simulink model "LCK"  (R2018b)
settings: Solver=FixedStepDiscrete  StartTime=0.0  StopTime=inf  FixedStep=0.01  RelTol=1e-3
PostLoadFcn:
  | if any(exist('dsrtsu_mdlpostloadfcn', 'file') ~= 0), dsrtsu_mdlpostloadfcn('Execute', bdroot); end
values from neighbouring files (symbols this model uses):
  C_DEG2RAD = 0.0175    [LCK_Macro.sldd]
  C_KPH2MPS = 0.2778    [LCK_Macro.sldd]
  C_NEARZERO = 0.0001    [LCK_Macro.sldd]
  C_ONE = 1.0    [LCK_Macro.sldd]
  C_RAD2DEG = 57.2958    [LCK_Macro.sldd]
  C_ZERO = 0.0    [LCK_Macro.sldd]
  k_accel_pedal_pos_per_speed_x : value not decoded    [LCK_LogicPara.sldd]
  k_accel_pedal_pos_per_speed_z : value not decoded    [LCK_LogicPara.sldd]
  k_brake_suprress_hold = 1000.0    [LCK_LogicPara.sldd]
  k_driver_appl_torque_filt = 50.0    [LCK_LogicPara.sldd]
  k_driver_suppression_hold_time = 3000.0    [LCK_LogicPara.sldd]
  k_hands_on_wheel_hold_msec = 500.0    [LCK_LogicPara.sldd]
  k_hands_on_wheel_torque_hi = 0.2    [LCK_LogicPara.sldd]
  k_hands_on_wheel_torque_lo = 0.15    [LCK_LogicPara.sldd]
  k_handsoff_delay_cycles = 50.0    [LCK_LogicPara.sldd]
  k_handsoff_torq_Lo_CR = 0.3    [LCK_LogicPara.sldd]
  k_handson_delay_cycles = 5.0    [LCK_LogicPara.sldd]
  k_HighAccel_suppress_hold = 3000.0    [LCK_LogicPara.sldd]
  k_HLR_suprress_hold = 3000.0    [LCK_LogicPara.sldd]
  k_hs_StrAng_CR_threshold_z : value not decoded    [LCK_LogicPara.sldd]
  k_LC_Exit_Switch = 0.0    [LCK_LogicPara.sldd]
  k_LCG_Configured = 1.0    [LCK_LogicPara.sldd]
  k_LCK_A0_Rdy2Act_UseConst = 0.0    [LCK_LogicPara.sldd]
  k_LCK_A0Fac_ActSta : value not decoded    [LCK_CtrlPara.sldd]
  k_LCK_A0Fac_DrvStm : value not decoded    [LCK_CtrlPara.sldd]
  k_LCK_A0Shift_LftCurv : value not decoded    [LCK_CtrlPara.sldd]
  k_LCK_A0Shift_RgtCurv : value not decoded    [LCK_CtrlPara.sldd]
  k_LCK_A0Shift_StraLan = 0.0    [LCK_CtrlPara.sldd]
  k_LCK_A0ShiftFac_Dy_LftCurv : value not decoded    [LCK_CtrlPara.sldd]
  k_LCK_A0ShiftFac_Dy_RgtCurv : value not decoded    [LCK_CtrlPara.sldd]
  k_LCK_A0ShiftFac_Vspd : value not decoded    [LCK_CtrlPara.sldd]
  k_LCK_accel_inhibit_thold = 35.0    [LCK_LogicPara.sldd]
  k_LCK_Active2Ready_Mask = 255.0    [LCK_LogicPara.sldd]
  k_LCK_CvatRateBks : value not decoded    [LCK_CtrlPara.sldd]
  k_LCK_CvatrBks : value not decoded    [LCK_CtrlPara.sldd]
  k_LCK_DFac_Dy : value not decoded    [LCK_CtrlPara.sldd]
  k_LCK_DFac_Dy_Curv : value not decoded    [LCK_CtrlPara.sldd]
  k_LCK_DFac_HaCurCen : value not decoded    [LCK_CtrlPara.sldd]
  k_LCK_DFac_HaCurSid : value not decoded    [LCK_CtrlPara.sldd]
  k_LCK_DFac_HadCurCen : value not decoded    [LCK_CtrlPara.sldd]
  k_LCK_DFac_HadCurSid : value not decoded    [LCK_CtrlPara.sldd]
  k_LCK_DFac_HadStrCen : value not decoded    [LCK_CtrlPara.sldd]
  k_LCK_DFac_HadStrSid : value not decoded    [LCK_CtrlPara.sldd]
  k_LCK_DFac_HaStrCen : value not decoded    [LCK_CtrlPara.sldd]
  k_LCK_DFac_HaStrSid : value not decoded    [LCK_CtrlPara.sldd]
  k_LCK_DFac_Rad : value not decoded    [LCK_CtrlPara.sldd]
  k_LCK_DFac_SA_CurCen : value not decoded    [LCK_CtrlPara.sldd]
  k_LCK_DFac_SA_CurSid : value not decoded    [LCK_CtrlPara.sldd]
  k_LCK_DFac_SA_StrCen : value not decoded    [LCK_CtrlPara.sldd]
  k_LCK_DFac_SA_StrSid : value not decoded    [LCK_CtrlPara.sldd]
  k_LCK_DFac_SS_CurCen : value not decoded    [LCK_CtrlPara.sldd]
  k_LCK_DFac_SS_CurSid : value not decoded    [LCK_CtrlPara.sldd]
  k_LCK_DFac_SS_StrCen : value not decoded    [LCK_CtrlPara.sldd]
  k_LCK_DFac_SS_StrSid : value not decoded    [LCK_CtrlPara.sldd]
  k_LCK_DFac_Vspd : value not decoded    [LCK_CtrlPara.sldd]
  k_LCK_DlyTm_DrvStim = 0.2    [LCK_CtrlPara.sldd]
  k_LCK_DTermMax = 2.0    [LCK_CtrlPara.sldd]
  k_LCK_DyBks_Curv : value not decoded    [LCK_CtrlPara.sldd]
  k_LCK_Enable_POOnly = 1.0    [LCK_LogicPara.sldd]
  k_LCK_Entry_DistBuffer = 0.1    [LCK_LogicPara.sldd]
  k_LCK_Fac_Vspd2RngThr_FalRec = 0.23    [LCK_CtrlPara.sldd]
  k_LCK_Ffw_CvatSwh = 0.0    [LCK_CtrlPara.sldd]
  k_LCK_Ffw_DyBks : value not decoded    [LCK_CtrlPara.sldd]
  k_LCK_Ffw_TimCon_CmdFlt = 0.0    [LCK_CtrlPara.sldd]
  k_LCK_FfwDeltaFac_Rad_Lft : value not decoded    [LCK_CtrlPara.sldd]
  k_LCK_FfwDeltaFac_Rad_Rgt : value not decoded    [LCK_CtrlPara.sldd]
  k_LCK_FfwDeltaFac_Vspd : value not decoded    [LCK_CtrlPara.sldd]
  k_LCK_FfwFac_CvatRate_Lft : value not decoded    [LCK_CtrlPara.sldd]
  k_LCK_FfwFac_CvatRate_Rgt : value not decoded    [LCK_CtrlPara.sldd]
  k_LCK_FfwFac_Dy : value not decoded    [LCK_CtrlPara.sldd]
  k_LCK_FfwFac_Rad_Lft : value not decoded    [LCK_CtrlPara.sldd]
  k_LCK_FfwFac_Rad_Rgt : value not decoded    [LCK_CtrlPara.sldd]
  k_LCK_FfwFac_Vspd : value not decoded    [LCK_CtrlPara.sldd]
  k_LCK_FfwTorq_Cvat : value not decoded    [LCK_CtrlPara.sldd]
  k_LCK_HAFac_ActSta : value not decoded    [LCK_CtrlPara.sldd]
  k_LCK_HAFac_DrvStm : value not decoded    [LCK_CtrlPara.sldd]
  k_LCK_HaloTime = 2000.0    [LCK_LogicPara.sldd]
  k_LCK_HaloTime_Switch = 0.0    [LCK_LogicPara.sldd]
  k_LCK_HARFac_ActSta : value not decoded    [LCK_CtrlPara.sldd]
  k_LCK_HARFac_DrvStm : value not decoded    [LCK_CtrlPara.sldd]
  k_LCK_Hed_DyBks : value not decoded    [LCK_CtrlPara.sldd]
  k_LCK_HedAngDiffX : value not decoded    [LCK_CtrlPara.sldd]
  k_LCK_HedAngRateDiffX : value not decoded    [LCK_CtrlPara.sldd]
  k_LCK_HndsOnWhel_DlyTm_Idl2Rdy = 0.0    [LCK_LogicPara.sldd]
  k_LCK_host_veh_width = 1.86    [LCK_LogicPara.sldd]
  k_LCK_Idle2Ready_Mask = 239.0    [LCK_LogicPara.sldd]
  k_LCK_Junc_SusTime = 1.0    [LCK_LogicPara.sldd]
  k_LCK_KpKdDecSlopeLmt = 10.0    [LCK_CtrlPara.sldd]
  k_LCK_KpKdIncSlopeLmt = 5.0    [LCK_CtrlPara.sldd]
  k_LCK_Lat_Ctrl_DFac_Lft = 1.0    [LCK_CtrlPara.sldd]
  k_LCK_Lat_Ctrl_DFac_Rgt = 1.05    [LCK_CtrlPara.sldd]
  k_LCK_Lat_Ctrl_Kd = 0.8    [LCK_CtrlPara.sldd]
  k_LCK_Lat_Ctrl_Ki = 0.5    [LCK_CtrlPara.sldd]
  k_LCK_Lat_Ctrl_Kp = 0.7    [LCK_CtrlPara.sldd]
  k_LCK_Lat_Ctrl_Kp_NearGain = 0.7    [LCK_CtrlPara.sldd]
  k_LCK_Lat_Ctrl_PFac_Lft = 1.0    [LCK_CtrlPara.sldd]
  k_LCK_Lat_Ctrl_PFac_Rgt = 1.05    [LCK_CtrlPara.sldd]
  k_LCK_Lat_Ctrl_TimCon_CmdFlt = 5.0    [LCK_CtrlPara.sldd]
  k_LCK_Lat_DFac_Rad : value not decoded    [LCK_CtrlPara.sldd]
  k_LCK_Lat_DFac_SS_Cur : value not decoded    [LCK_CtrlPara.sldd]
  k_LCK_Lat_DFac_SS_Str : value not decoded    [LCK_CtrlPara.sldd]
  k_LCK_Lat_DFac_Vspd : value not decoded    [LCK_CtrlPara.sldd]
  k_LCK_Lat_DyBks : value not decoded    [LCK_CtrlPara.sldd]
  k_LCK_Lat_IFac_Rad : value not decoded    [LCK_CtrlPara.sldd]
  k_LCK_Lat_IFac_Vspd : value not decoded    [LCK_CtrlPara.sldd]
  k_LCK_Lat_ILmtFac_Dy_CurvLan : value not decoded    [LCK_CtrlPara.sldd]
  k_LCK_Lat_ILmtFac_Dy_StraLan : value not decoded    [LCK_CtrlPara.sldd]
  k_LCK_Lat_ILmtFac_Rad : value not decoded    [LCK_CtrlPara.sldd]
  k_LCK_Lat_ILmtFac_Rad_NearGain = 1.0    [LCK_CtrlPara.sldd]
  k_LCK_Lat_ILmtFac_Vspd_CurvLan : value not decoded    [LCK_CtrlPara.sldd]
  k_LCK_Lat_ILmtFac_Vspd_StraLan : value not decoded    [LCK_CtrlPara.sldd]
  k_LCK_Lat_ITermLmt_Dy = 1.0    [LCK_CtrlPara.sldd]
  k_LCK_Lat_KpKdDecSlopeLmt = 10.0    [LCK_CtrlPara.sldd]
  k_LCK_Lat_KpKdIncSlopeLmt = 10.0    [LCK_CtrlPara.sldd]
  k_LCK_Lat_PFac_Dy_InnLftCur : value not decoded    [LCK_CtrlPara.sldd]
  k_LCK_Lat_PFac_Dy_InnRgtCur : value not decoded    [LCK_CtrlPara.sldd]
  k_LCK_Lat_PFac_Dy_OutLftCur : value not decoded    [LCK_CtrlPara.sldd]
  k_LCK_Lat_PFac_Dy_OutRgtCur : value not decoded    [LCK_CtrlPara.sldd]
  k_LCK_Lat_PFac_Dy_Str : value not decoded    [LCK_CtrlPara.sldd]
  k_LCK_Lat_PFac_Rad : value not decoded    [LCK_CtrlPara.sldd]
  ... (+153 more)
undefined symbols (not defined in the file or in its folder): k_LCK_CurvBks, K_LCK_SPA0A1A2_LMRngCmp_y
libraries: LateralControl_fcns_lib x59, simulink x24
(part 1 of 47)
settings Model: DSRTSU_INTERNAL_RTI_VER=540  DSRTSU_INTERNAL_RTI_TYPE=rti1401  RTICANMMDATA=struct('GeneralSetupData',struct('modelroot','D:\0001_SAIC_MBD\03_ZOP\ZOP_Integration\ZOP_Integration_AVP','generalsettings',struct('filesettings',struct('destfolder',struct('Name','RTICANMM_FILES','Check',1),'buildfolder',struct('Name','.','Check',1),'AbsDestfolder',struct('Name','D:\0001_SAIC_MBD\03_ZOP\ZOP_Integration\ZOP_Integration_AVP\RTICANMM_FILES'),'AbsBuildfolder',struct('Name','D:\0001_SAIC_MBD\03_ZOP\ZOP_Integration\ZOP_Integration_AVP'))),'options',struct('addpaths',1,'rmpaths',1,'addtrcexclusion',logical(1),'cannavigator',struct('checkmonitoring',0),'show_usrtrc',0,'use_usrtrc',0),'advanced',struct('options',ones(1,100)),'MPSetup',{{}},'RTI',struct('Type','RTI1401','Ver','7.12','Date','02-May-2019'),'modelname','LCK','block','LCK'))  DSRTSU_INTERNAL_RTIFPGA=130  Creator=chenx  LastModifiedBy=qiand
settings OptimizationCC: BlockReduction=off  ConditionallyExecuteInputs=off  DefaultUnderspecifiedDataType=single  BufferReuse=off  EnhancedBackFolding=on  ExpressionFolding=off  PassReuseOutputArgsThreshold=0  LocalBlockOutputs=off  OptimizeBlockOrder=speed  DifferentSizesBufferReuse=on
settings DebuggingCC: ParameterTunabilityLossMsg=error  UnderSpecifiedDimensionMsg=warning
settings HardwareCC: ProdBitPerPointer=32  ProdBitPerSizeT=32  ProdBitPerPtrDiffT=32  ProdLargestAtomicInteger=Integer  ProdEndianess=BigEndian  ProdWordSize=32  ProdHWDeviceType=Custom Processor->Custom  TargetIntDivRoundTo=Zero  TargetEndianess=BigEndian  TargetHWDeviceType=Custom Processor->Custom
settings ModelReferenceCC: ModelReferenceNumInstancesAllowed=Single
settings SFSimCC: MATLABDynamicMemAlloc=off
settings RTWCC: SystemTargetFile=rti1401.tlc  MakeCommand=make_rti  TemplateMakefile=rti1401.tmf  Description=dSPACE DS1401 Hardware Platform  GenerateReport=on  LaunchReport=on
settings CodeAppCC: OperatorAnnotations=on
settings STFCustomTargetCC: ParMdlRefBuildCompliant=on  SystemTargetFile=rti1401.tlc
settings GRTTargetCC: TargetLangStandard=C89/C90 (ANSI)  CompOptLevelCompliant=off  ConcurrentExecutionCompliant=off  CombineOutputUpdateFcns=off  MatFileLogging=off  CPPClassGenCompliant=off  UseToolchainInfoCompliant=off

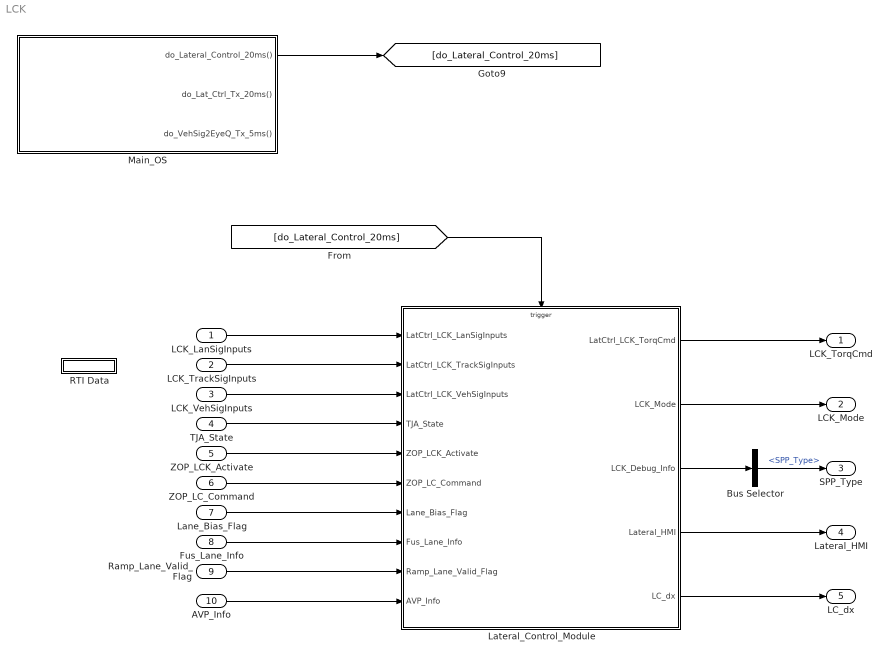
== system LCK ==
  LCK_LanSigInputs : Inport  OutDataTypeStr=Bus: LatCtrl_LCK_LanSigInputs_t  BusOutputAsStruct=on
  LCK_TrackSigInputs : Inport  Port=2  OutDataTypeStr=Bus: LatCtrl_LCK_TrackSigInputs_t  BusOutputAsStruct=on
  LCK_VehSigInputs : Inport  Port=3  OutDataTypeStr=Bus: LatCtrl_LCK_VehSigInputs_t  BusOutputAsStruct=on
  TJA_State : Inport  Description=_GWMAB30P4.LCK.000_80_  Port=4
  ZOP_LCK_Activate : Inport  Description=_GWMAB30P4.LCK.000_80_  Port=5
  ZOP_LC_Command : Inport  Port=6
  Lane_Bias_Flag : Inport  Port=7
  Fus_Lane_Info : Inport  Description=_GWMH9P3.Latctrl.000_23_  Port=8  OutDataTypeStr=Bus: FUS_LANE_OUTPUT_ST
  Ramp_Lane_Valid_Flag : Inport  Port=9
  AVP_Info : Inport  Port=10  OutDataTypeStr=Bus: AVP_OUTPUT_ST  BusOutputAsStruct=on
  Bus Selector : BusSelector  OutputSignals=SPP_Info.SPP_Type
  Lateral_Control_Module : Subsystem
  Main_OS : Stateflow chart  TreatAsAtomicUnit=on
  RTI Data : Subsystem  Tag=struct('RTIDataServer',struct('RTIDataServerVs','2','RTIModelDescription','struct(''main'',''LCK'',''sub'','''',''isMp'',0)'))  LoadFcn="if exist('rtidc'), try,  rtidc('DataHostBlockClbLoad', gcbh); catch, disp(['Warning: ''LoadFcn'' for RTI Data block failed: ' lasterr]); end, end,"  mask(RTI_DATA_HOST){}
      mask help:
      | RTI Data Block.
      | This block is used by RTI to store internal model-dependent data.
      | Please keep this block on the root level of the model. Deleting this block will result in data loss.
      |
      | NEVER DELETE OR COPY THIS BLOCK!
      settings: CopyFcn="if exist('rtidc'), try,  rtidc('DataHostBlockClbCopy', gcbh); catch, disp(['Warning: ''CopyFcn'' for RTI Data block failed: ' lasterr]); end, end,"  DeleteFcn="if exist('rtidc'), try,  rtidc('DataHostBlockClbDelete', gcbh); catch, disp(['Warning: ''DeleteFcn'' for RTI Data block failed: ' lasterr]); end, end,"  ModelCloseFcn="if exist('rtidc'), try,  rtidc('DataHostBlockClbModelClose', gcbh); catch, disp(['Warning: ''ModelCloseFcn'' for RTI Data block failed: ' lasterr]); end, end,"  PreSaveFcn="if exist('rtidc'), try,  rtidc('DataHostBlockClbPreSave', gcbh); catch, disp(['Warning: ''PreSaveFcn'' for RTI Data block failed: ' lasterr]); end, end,"  PostSaveFcn="if exist('rtidc'), try,  rtidc('DataHostBlockClbPostSave', gcbh); catch, disp(['Warning: ''PostSaveFcn'' for RTI Data block failed: ' lasterr]); end, end,"  NameChangeFcn="if exist('rtidc'), try,  rtidc('DataHostBlockClbNameChange', gcbh); catch, disp(['Warning: ''NameChangeFcn'' for RTI Data block failed: ' lasterr]); end, end,"
      mask Help:
      | RTI Data Block.
      | This block is used by RTI to store internal model-dependent data.
      | Please keep this block on the root level of the model. Deleting this block will result in data loss.
      | 
      | NEVER DELETE OR COPY THIS BLOCK!
      mask Display:
      | text(0.5, 0.5, 'RTI Data', 'HorizontalAlignment', 'center');
      | plot([1 0]);
  LCK_TorqCmd : Outport
  LCK_Mode : Outport  Port=2
  SPP_Type : Outport  Port=3
  Lateral_HMI : Outport  Description=_GWMAB30P4.LCK.000_194_  Port=4  OutDataTypeStr=Bus: HMI_Lateral_t
  LC_dx : Outport  Port=5
  wires:
  LCK_LanSigInputs/1 -> Lateral_Control_Module/1(LatCtrl_LCK_LanSigInputs)
  LCK_TrackSigInputs/1 -> Lateral_Control_Module/2(LatCtrl_LCK_TrackSigInputs)
  LCK_VehSigInputs/1 -> Lateral_Control_Module/3(LatCtrl_LCK_VehSigInputs)
  Lateral_Control_Module/1(LatCtrl_LCK_TorqCmd) -> LCK_TorqCmd/1
  Lateral_Control_Module/2(LCK_Mode) -> LCK_Mode/1
  Main_OS/1(do_Lateral_Control_20ms()) -> [do_Lateral_Control_20ms]
  [do_Lateral_Control_20ms] -> Lateral_Control_Module/Trigger
  Lateral_Control_Module/3(LCK_Debug_Info) -> Bus Selector/1
  Bus Selector/1 -> SPP_Type/1  "<SPP_Type>"
  Lateral_Control_Module/4(Lateral_HMI) -> Lateral_HMI/1
  TJA_State/1 -> Lateral_Control_Module/4(TJA_State)
  ZOP_LCK_Activate/1 -> Lateral_Control_Module/5(ZOP_LCK_Activate)
  ZOP_LC_Command/1 -> Lateral_Control_Module/6(ZOP_LC_Command)
  Lateral_Control_Module/5(LC_dx) -> LC_dx/1
  Lane_Bias_Flag/1 -> Lateral_Control_Module/7(Lane_Bias_Flag)
  Fus_Lane_Info/1 -> Lateral_Control_Module/8(Fus_Lane_Info)
  Ramp_Lane_Valid_Flag/1 -> Lateral_Control_Module/9(Ramp_Lane_Valid_Flag)
  AVP_Info/1 -> Lateral_Control_Module/10(AVP_Info)

== system LCK/Lateral_Control_Module ==
  LatCtrl_LCK_LanSigInputs : Inport  OutDataTypeStr=Bus: LatCtrl_LCK_LanSigInputs_t
  LatCtrl_LCK_TrackSigInputs : Inport  Description=_GWMAB30P4.LCK.000_220_  Port=2  OutDataTypeStr=Bus: LatCtrl_LCK_TrackSigInputs_t
  LatCtrl_LCK_VehSigInputs : Inport  Description=_GWMAB30P4.LCK.000_287_  Port=3  OutDataTypeStr=Bus: LatCtrl_LCK_VehSigInputs_t
  TJA_State : Inport  Description=_GWMAB30P4.LCK.000_80_  Port=4
  ZOP_LCK_Activate : Inport  Description=_GWMAB30P4.LCK.000_80_  Port=5
  ZOP_LC_Command : Inport  Port=6
  Lane_Bias_Flag : Inport  Port=7
  Fus_Lane_Info : Inport  Description=_GWMH9P3.Latctrl.000_23_  Port=8
  Ramp_Lane_Valid_Flag : Inport  Port=9
  AVP_Info : Inport  Port=10  OutDataTypeStr=Bus: AVP_OUTPUT_ST  BusOutputAsStruct=on
  20msCall : TriggerPort  TriggerType=function-call  VariantControl=(inherit)
  Adas_Lateral_Control_LCK_Core : Subsystem
  Bus Creator : BusCreator  Inputs=4
  Bus Creator1 : BusCreator  Inputs=4
  Constant : Constant  Value=4
  LCK_State_Ctrl : Subsystem
  LC_Path_Process : Subsystem
  Lat_HMI : Subsystem
  Steer_Path_Process : Subsystem
  Switch : Switch  Criteria=u2 > Threshold  Threshold=0.5
  LatCtrl_LCK_TorqCmd : Outport
  LCK_Mode : Outport  Port=2
  LCK_Debug_Info : Outport  Description=_GWMAB30P4.LCK.000_194_  Port=3
  Lateral_HMI : Outport  Description=_GWMAB30P4.LCK.000_194_  Port=4  OutDataTypeStr=Bus: HMI_Lateral_t
  LC_dx : Outport  Port=5
  wires:
  Adas_Lateral_Control_LCK_Core/2(LatCtrl_LCK_TorqCmd) -> [LatCtrl_LCK_TorqCmd], LatCtrl_LCK_TorqCmd/1
  LatCtrl_LCK_TrackSigInputs/1 -> Adas_Lateral_Control_LCK_Core/4(LatCtrl_LCK_TrackSigInputs)
  Bus Creator/1 -> LCK_Debug_Info/1
  Adas_Lateral_Control_LCK_Core/1(LCK_Ctrl_Info) -> Bus Creator/1  "LCK_Ctrl_Info"
  LCK_State_Ctrl/2(LCK_State_Info) -> [LCK_State_Info]
  LatCtrl_LCK_LanSigInputs/1 -> [LanSigInputs], LC_Path_Process/1(LatCtrl_LCK_LanSigInputs), LCK_State_Ctrl/1(LatCtrl_LCK_LanSigInputs), Adas_Lateral_Control_LCK_Core/2(LatCtrl_LCK_LanSigInputs), Steer_Path_Process/1(Vis_Lane_Info)
  LatCtrl_LCK_VehSigInputs/1 -> Steer_Path_Process/7(LatCtrl_LCK_VehSigInputs), Adas_Lateral_Control_LCK_Core/3(LatCtrl_LCK_VehSigInputs), LC_Path_Process/2(LatCtrl_LCK_VehSigInputs), LCK_State_Ctrl/2(LatCtrl_LCK_VehSigInputs)
  Steer_Path_Process/1(SPP_Info) -> Adas_Lateral_Control_LCK_Core/1(LatCtrl_LCK_SPPInfo), [SPP_Info]
  [SPP_Info] -> LCK_State_Ctrl/3(LatCtrl_LCK_SPPInfo)
  [LCK_Mode] -> Steer_Path_Process/2(LCK_Mode)
  [SPP_Info] -> Bus Creator/3  "SPP_Info"
  [LanSigInputs] -> Bus Creator/4  "LanSigInputs"
  [LCK_State_Info] -> Bus Creator/2  "LCK_State_Info"
  [LatCtrl_LCK_TorqCmd] -> LCK_State_Ctrl/4(Final_Torq_Cmd)
  [LCK_Mode] -> Lat_HMI/2(LCK_Mode)
  LCK_State_Ctrl/3(Driver_Operation_Info) -> Lat_HMI/1(Driver_Operation_Info)
  Lat_HMI/1(Lateral_HMI) -> Lateral_HMI/1
  [SPP_Info] -> LC_Path_Process/3(SPP_Info)  "SPP_Info"
  [LCK_Mode] -> LC_Path_Process/4(LCK_Mode)
  LC_Path_Process/1(LC_A0) -> Bus Creator1/1
  LC_Path_Process/2(LC_A1) -> Bus Creator1/2
  LC_Path_Process/3(LC_A2) -> Bus Creator1/3
  Bus Creator1/1 -> [LC_Info]
  [LC_Info] -> Adas_Lateral_Control_LCK_Core/6(LC_Info)
  LC_Path_Process/4(LC_Phase) -> Bus Creator1/4
  [LC_Info] -> LCK_State_Ctrl/5(LC_Info)
  TJA_State/1 -> LCK_State_Ctrl/6(TJA_State)
  ZOP_LCK_Activate/1 -> LCK_State_Ctrl/7(ZOP_LCK_Activate)
  ZOP_LC_Command/1 -> [ZOP_LC_Command], LCK_State_Ctrl/8(ZOP_LC_Command)
  LC_Path_Process/5(LC_dx) -> LC_dx/1, Lat_HMI/4(LC_dx)
  Fus_Lane_Info/1 -> Steer_Path_Process/3(Fus_Lane_Info)
  Lane_Bias_Flag/1 -> Steer_Path_Process/4(Lane_Bias_Flag)
  [ZOP_LC_Command] -> Lat_HMI/3(ZOP_LC_Command)
  LC_Path_Process/6(LC_dy) -> Lat_HMI/5(LC_dy)
  Steer_Path_Process/2(PO_Enable) -> [PO_Enable]
  [PO_Enable] -> LCK_State_Ctrl/9(PO_Enable)
  Ramp_Lane_Valid_Flag/1 -> Steer_Path_Process/5(Ramp_Lane_Valid_Flag)
  AVP_Info/1 -> Steer_Path_Process/6(AVP_Info)
  Steer_Path_Process/3(AVP_Enable) -> [AVP_Enable]
  LCK_State_Ctrl/1(LCK_Mode) -> Switch/3, LCK_Mode/1, [LCK_Mode]
  Switch/1 -> Adas_Lateral_Control_LCK_Core/5(LatCtrl_LCK_LogicSigInputs)
  [AVP_Enable] -> Switch/2
  Constant/1 -> Switch/1
  [AVP_Enable] -> Adas_Lateral_Control_LCK_Core/7(AVP_Enable)

== system LCK/RTI Data ==
  RTI Data Store : Subsystem  Tag="struct('private',struct('version',struct('dsVer',uint32(2),'dsVerCreation',uint32(2),'RTI',struct('ver','7.12','type','RTI1401')),'access',struct('type','Model','isPerm',1,'created',['11-Dec-2020 17:36:09'],'modified',['16-Mar-2021 19:09:48'],'location','')),'public',struct('main',struct('data',[]),'sub',struct('name',{{'LCK'}},'data',{{struct('TH',struct('thTaskInfo',struct('taskType',{'TIMER','HWINT','TMRINT','SWINT','GLINT'},'tasksNumOf',{1,0,0,0,0},'srcIds',{{'TIMERA'},{},{},{},{}},'taskNames',{{['Timer Task 1']},{},{},{},{}})),'th_tc',struct('dataType','TASK','taskGroupId','','taskGroupList',{{}},'taskSchedulingPolicy','FCFS','taskType','TIMER','blkh',-1,'srcId','TIMERA','srcSgnName',['Timer A interrupt'],'srcCpuName','','taskName',['Timer Task 1  [0.01] s'],'taskNameDisplayExt','','smplTime',0.01,'smplTimeOffs',0,'hasFixedPriority',0,'priority',1,'hasFixedOvc',0,'ovcType',1,'ovcMax',1),'tc_th',struct('dataType','TASK','taskGroupId','','taskGroupList',{{}},'taskSchedulingPolicy','FCFS','taskType','TIMER','blkh',-1,'srcId','TIMERA','srcSgnName',['Timer A interrupt'],'srcCpuName','','taskName',['Timer Task 1  [0.01] s'],'taskNameDisplayExt','','smplTime',0.01,'smplTimeOffs',0,'hasFixedPriority',0,'priority',1,'hasFixedOvc',0,'ovcType',1,'ovcMax',1))}})))"  mask(RTI_DATA_STORE){}
      mask help:
      | RTI Data Store Block. This block is used by RTI to store internal model dependent data. Deleting this block will result in data loss.
      |
      | NEVER DELETE, COPY, OR MODIFY THIS BLOCK!
      mask Help:
      | RTI Data Store Block. This block is used by RTI to store internal model dependent data. Deleting this block will result in data loss.
      | 
      | NEVER DELETE, COPY, OR MODIFY THIS BLOCK!
      mask Display: text(0.5, 0.5, ' ', 'HorizontalAlignment', 'center');
